simulink model "GreenCraneSimulator_SomplifiedHydMechModel"  (R2021b)
settings: Solver=ode23  StartTime=0.0  StopTime=25  FixedStep=0.0001  RelTol=1e-3
undefined symbols (not defined in the file): DiscIntNeverNeededParam, tCycle, X, Y, Z
libraries: sm_lib x25, nesl_utility x4, simulink x1
(part 2 of 2)

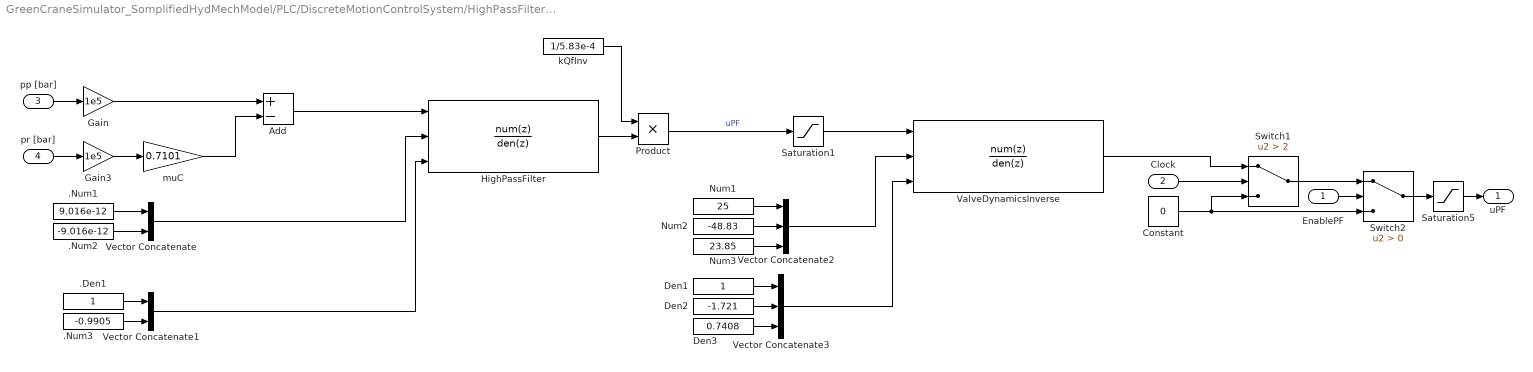
== system GreenCraneSimulator_SomplifiedHydMechModel/PLC/DiscreteMotionControlSystem/HighPassFilteredPressureFeedback (PF) ==
  EnablePF : Inport  OutDataTypeStr=boolean
  Clock : Inport  Port=2
  pp [bar] : Inport  Port=3
  pr [bar] : Inport  Port=4
  .Den1 : Constant
  .Num1 : Constant  Value=9.016e-12
  .Num2 : Constant  Value=-9.016e-12
  .Num3 : Constant  Value=-0.9905
  Add : Sum  Inputs=+-
  Constant : Constant  Value=0
  Den1 : Constant
  Den2 : Constant  Value=-1.721
  Den3 : Constant  Value=0.7408
  Gain : Gain  Gain=1e5
  Gain3 : Gain  Gain=1e5
  HighPassFilter : DiscreteTransferFcn  NumeratorSource=Input port  Numerator=[3.786e-11 -3.786e-11]  DenominatorSource=Input port  Denominator=[1 -0.9954]  a0EqualsOne=on
      settings: InputPortMap=u0,p1,p3
  Num1 : Constant  Value=25
  Num2 : Constant  Value=-48.83
  Num3 : Constant  Value=23.85
  Product : Product
  Saturation1 : Saturate  UpperLimit=1  LowerLimit=-1
  Saturation5 : Saturate  UpperLimit=1  LowerLimit=-1
  Switch1 : Switch  Criteria=u2 > Threshold  Threshold=2
  Switch2 : Switch  Criteria=u2 > Threshold
  ValveDynamicsInverse : DiscreteTransferFcn  NumeratorSource=Input port  Numerator=[25 -48.83 23.85]  DenominatorSource=Input port  Denominator=[1 -1.721 0.7408]  a0EqualsOne=on
      settings: InputPortMap=u0,p1,p3
  Vector Concatenate : Concatenate
  Vector Concatenate1 : Concatenate
  Vector Concatenate2 : Concatenate  NumInputs=3
  Vector Concatenate3 : Concatenate  NumInputs=3
  kQfInv : Constant  Value=1/5.83e-4
  muC : Gain  Gain=0.7101
  uPF : Outport  VectorParamsAs1DForOutWhenUnconnected=off
  wires:
  pr [bar]/1 -> Gain3/1
  pp [bar]/1 -> Gain/1
  Add/1 -> HighPassFilter/1
  Gain/1 -> Add/1
  HighPassFilter/1 -> Product/2
  Constant/1 -> Switch1/3, Switch2/3
  Gain3/1 -> muC/1
  Vector Concatenate/1 -> HighPassFilter/2
  Vector Concatenate1/1 -> HighPassFilter/3
  .Num1/1 -> Vector Concatenate/1
  .Num2/1 -> Vector Concatenate/2
  .Den1/1 -> Vector Concatenate1/1
  .Num3/1 -> Vector Concatenate1/2
  Switch2/1 -> Saturation5/1
  Switch1/1 -> Switch2/1
  EnablePF/1 -> Switch2/2
  Saturation5/1 -> uPF/1
  Vector Concatenate2/1 -> ValveDynamicsInverse/2
  Vector Concatenate3/1 -> ValveDynamicsInverse/3
  Den1/1 -> Vector Concatenate3/1
  Den2/1 -> Vector Concatenate3/2
  Den3/1 -> Vector Concatenate3/3
  ValveDynamicsInverse/1 -> Switch1/1
  kQfInv/1 -> Product/1
  muC/1 -> Add/2
  Num1/1 -> Vector Concatenate2/1
  Num2/1 -> Vector Concatenate2/2
  Num3/1 -> Vector Concatenate2/3
  Saturation1/1 -> ValveDynamicsInverse/1
  Product/1 -> Saturation1/1  "uPF"
  Clock/1 -> Switch1/2

== matlab function GreenCraneSimulator_SomplifiedHydMechModel/PLC/DiscreteMotionControlSystem/FB_ResetIntegralController/ResetIntegralController ==
  data: vRef input; exCylMax input; Reset output; exCyl input
function Reset = fcn(vRef, exCylMax, exCyl)

if abs(vRef) > 0 || abs(exCyl) > exCylMax
Reset = 0;
else 
Reset = 1;
end

== matlab function GreenCraneSimulator_SomplifiedHydMechModel/PLC/MotionReferenceTime/MATLAB Function ==
  data: StartClock input; StopClock input; Time output; Clock input
function Time = fcn(StartClock, StopClock, Clock)

if StartClock == 1 && ~StopClock
Time = Clock;
else
Time = 0.0;     
end

== matlab function GreenCraneSimulator_SomplifiedHydMechModel/PLC/CylinderDiscplacementToBoomAngle ==
  data: thetaBoom output; xCyl input
function thetaBoom  = fcn(xCyl)

%% Geomtry Constants
ABx = 0.427;
ABy = 1.057;
ACx = 0.49484;
ACy = 0.133;

AB = sqrt(abs(ABx)^2 + abs(ABy)^2);
AC = sqrt(abs(ACx)^2 + abs(ACy)^2);

BC = 0.77222 + xCyl;

alpha1 = atan(abs(ACy)/abs(ACx));
alpha2 = atan(abs(ABy)/abs(ABx));

theta1 = acos( (abs(AB)^2 + abs(AC)^2 - (abs(BC))^2) / (2 * abs(AB) * abs(AC)) ) - alpha2 + alpha1;

thetaBoom = theta1;

== matlab function GreenCraneSimulator_SomplifiedHydMechModel/PLC/MotionRefSelector/MATLAB Function ==
  data: AutoMode input; VelRef output; VelRefAuto input; PosRefAuto input; VelRefMan input; PosRef output; VFF output; PFC output
function [VelRef, PosRef, VFF, PFC] = fcn(AutoMode, VelRefAuto, PosRefAuto, VelRefMan)
if AutoMode == 1 
VelRef = VelRefAuto;
PosRef = PosRefAuto;
VFF = 1; 
PFC = 1; 
else 
VelRef = VelRefMan;
PosRef = 0.0;
VFF = 1; 
PFC = 0; 
end

== matlab function GreenCraneSimulator_SomplifiedHydMechModel/CraneSimulator/MATLAB Function ==
  data: uDCV input; xDot input; xDotDot output; x input; pPiston input; pRod input; pPistonDot output; pRodDot output
function [xDotDot, pPistonDot, pRodDot] = fcn(uDCV, xDot, x, pPiston, pRod)
%% Parameters
Fexternal = 1.3365e+04; % [N]
mEffective = 1.3365e+04;  % [kg]
kFric = 4000; % [N/(ms)]
Apiston = 0.0033; % [m^2]
Aannulus = 0.0023; % [m^2]
beta = 1.0e9; % [Pa]
pSupply = 180e5; % [Pa]
pReturn = 1.1e5; % [Pa]
MaxStroke = 0.5; % [m]
VCyl_A = 1.0e-03; 
VCyl_B = 1.25e-03; 
p_nom_DCV = 7e5;  
Q1_ref_DCV = 20/6e4;
kv1_DCV = Q1_ref_DCV/sqrt(p_nom_DCV);
p0 = 7e5; %compensator crack pressure
%% Directional Control Valve - Lifting Cylinder 
% LS Pressure
if uDCV > 0 
     pLS = pPiston;
 elseif uDCV < 0
     pLS = pRod;
 else 
     pLS = 0;
end
 
if pLS<0
    pLS = 0;
end

% Pressure Compensator
pPC = 0;

if p0 <= (pSupply - pLS) 
      pPC = pLS+p0; 
  elseif 0 < (pSupply - pLS) < p0
        pPC = pSupply-pLS;   
  elseif (pSupply - pLS) <= 0     
      pPC = pLS;
end

 if pPC<0
     pPC = 0;
 end
% Orifice Equations
if uDCV > 0
QDCV_in =  kv1_DCV*uDCV*sign(pPC-pPiston)*sqrt(abs(pPC-pPiston));
QDCV_out = kv1_DCV*uDCV*sign(pRod-pReturn)*sqrt(abs(pRod-pReturn));
elseif uDCV < 0  
QDCV_out =  kv1_DCV*uDCV*sign(pPC-pRod)*sqrt(abs(pPC-pRod));
QDCV_in =  kv1_DCV*uDCV*sign(pRod-pReturn)*sqrt(abs(pRod-pReturn));
else
QDCV_in = 0;
QDCV_out = 0;
end
%% Pressure Gradients
VA = VCyl_A + x*Apiston;
VB =  VCyl_B + (MaxStroke - x)*Aannulus; 
VA_dot = Apiston*xDot;
VB_dot = -Aannulus*xDot;
pPistonDot = beta/VA*(QDCV_in - VA_dot);
pRodDot = beta/VB*(-QDCV_out - VB_dot);

% Viscouse Friction
Ffric = kFric*xDot;

%% Hydraulic Force
Fhyd = pPiston*Apiston - pRod*Aannulus;

%% Newton Second Law of Motion
xDotDot = (Fhyd - Ffric - Fexternal)/mEffective;

== matlab function GreenCraneSimulator_SomplifiedHydMechModel/PLC/RampMotionProfileGenerator/RampSignal ==
  data: x0 input; v0 input; x_ref input; x output; v_ref input; t0 input; tRamp input; tWait input; v output; t input; T output; Error output
function [x,v,T, Error] = fcn(x0,v0, x_ref,v_ref,t0,tRamp,tWait,t)
x_SP = x_ref - x0;
vs=v_ref;
slopeExt=v0-vs;
slopeRetr=-vs-v0;

as = vs/tRamp;
s_acc=(vs^2-v0^2)/as;

tHold=(x_SP-s_acc)/vs;

if tHold < 0 
Error = 1;
else 
Error = 0;
end

t1=tRamp;
t2=tHold; 
t3=tRamp;
t4=tWait;
t5=t1;
t6=t2;
t7=t3;

x1 = x0 + v0*((t0+t1)-t0)-(slopeExt/t1)*((t0+t1)-t0)^2/2;
x2 = x1 + vs*((t0+t1+t2)-(t0+t1)); 
x4 = x_ref - v0*((t0+t1+t2+t3+t4+t5)-(t0+t1+t2+t3+t4))+(slopeRetr/t5)*((t0+t1+t2+t3+t4+t5)-(t0+t1+t2+t3+t4))^2/2; 
x5 = x4-vs*((t0+t1+t2+t3+t4+t5+t6)-(t0+t1+t2+t3+t4+t5));  

if Error == 1
x = x0;
v = v0; 
elseif t>=0 && t<t0
x = x0; 
v = v0;
elseif t>=t0 && t<(t0+t1)
x = x0 + v0*(t-t0)-(slopeExt/t1)*(t-t0)^2/2;
v = v0-(slopeExt/t1)*(t-t0);  
elseif t>=(t0+t1) && t<(t0+t1+t2)
x = x1 + vs*(t-(t0+t1)); 
v = vs; 
elseif t>=(t0+t1+t2) && t<(t0+t1+t2+t3)
x = x2+vs*(t-(t0+t1+t2))+(slopeExt/t3)*(t-(t0+t1+t2))^2/2; 
v = vs+(slopeExt/t3)*(t-(t0+t1+t2));   
elseif t>=(t0+t1+t2+t3) && t<(t0+t1+t2+t3+t4)
x = x_ref;
v = v0;  
elseif t>=(t0+t1+t2+t3+t4) && t<(t0+t1+t2+t3+t4+t5)
x = x_ref - v0*(t-(t0+t1+t2+t3+t4))+(slopeRetr/t5)*(t-(t0+t1+t2+t3+t4))^2/2; 
v = v0+(slopeRetr/t5)*(t-(t0+t1+t2+t3+t4));     
elseif t>=(t0+t1+t2+t3+t4+t5) && t<(t0+t1+t2+t3+t4+t5+t6)
x = x4-vs*(t-(t0+t1+t2+t3+t4+t5));   
v = -vs;    
elseif t>=(t0+t1+t2+t3+t4+t5+t6) && t<(t0+t1+t2+t3+t4+t5+t6+t7)
x = x5-vs*(t-(t0+t1+t2+t3+t4+t5+t6))-(slopeRetr/t3)*(t-(t0+t1+t2+t3+t4+t5+t6))^2/2;    
v = -vs-(slopeRetr/t3)*(t-(t0+t1+t2+t3+t4+t5+t6));     
else 
x = x0;
v = v0; 
end

T = t0+t1+t2+t3+t4+t5+t6+t7;
